simulink model "mot_sim"  (Simulink 4.00)
settings: Solver=ode45  SolverMode=SingleTasking  StartTime=0.0  StopTime=3  MaxStep=0.1  RelTol=1e-3  AbsTol=1e-3
values from neighbouring files (symbols this model uses):
  b = 0.1    [MOTOR.M]
  J = 0.01    [MOTOR.M]
  K = 0.01    [MOTOR.M]
  L = 0.5    [MOTOR.M]
  R = 1    [MOTOR.M]
settings Model: LastModifiedBy=R.Babuska  SaveTime=off  SaveOutput=off  LimitDataPoints=off  RTWTemplateMakefile=grt_vc.tmf

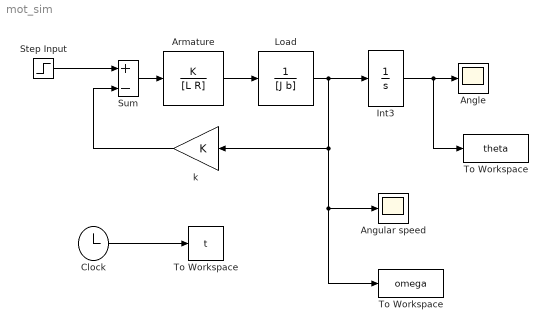
== system mot_sim ==
  " k " : Gain  Orientation=left  Gain=K  Multiplication=Element-wise(K.*u)  SaturateOnIntegerOverflow=on
  Angle : Scope
      settings: TickLabels=on  TimeRange=auto  YMin=0  YMax=0.5  SaveToWorkspace=off  SaveName=ScopeData  DataFormat=Array  LimitDataPoints=on  MaxDataPoints=5000
  Angular speed : Scope
      settings: TickLabels=on  TimeRange=auto  YMin=0  YMax=0.2  SaveToWorkspace=off  SaveName=ScopeData  DataFormat=Array  LimitDataPoints=on  MaxDataPoints=5000
  Armature : TransferFcn  Numerator=K  Denominator=[L R]  AbsoluteTolerance=auto  Realization=auto
  Clock : Clock
      settings: DisplayTime=off  Decimation=10
  Int3 : Integrator  ExternalReset=none  InitialConditionSource=internal  InitialCondition=0  LimitOutput=off  UpperSaturationLimit=inf  LowerSaturationLimit=-inf  ShowSaturationPort=off  ShowStatePort=off  AbsoluteTolerance=auto
  Load : TransferFcn  Numerator=1  Denominator=[J b]  AbsoluteTolerance=auto  Realization=auto
  Step Input : Step  Time=0  Before=0  After=1  SampleTime=-1
  Sum : Sum  Inputs=+-  SaturateOnIntegerOverflow=on
  To Workspace : ToWorkspace  VariableName=omega  SampleTime=0  SaveFormat=Array
      settings: MaxDataPoints=1000
  "To Workspace " : ToWorkspace  VariableName=theta  SampleTime=0  SaveFormat=Array
      settings: MaxDataPoints=1000
  "To Workspace  " : ToWorkspace  VariableName=t  SampleTime=0  SaveFormat=Array
      settings: MaxDataPoints=1000
  wires:
  Sum/1 -> Armature/1
  Armature/1 -> Load/1
  Load/1 -> Int3/1, " k "/1, Angular speed/1, To Workspace/1
  " k "/1 -> Sum/2
  Int3/1 -> Angle/1, "To Workspace "/1
  Step Input/1 -> Sum/1
  Clock/1 -> "To Workspace  "/1
